simulink library "INT_ECBtn_DD"  (R2016b)
settings: Solver=VariableStepAuto  StartTime=0.0  StopTime=10.0  RelTol=1e-3
settings Model: Creator=xinchangran  LastModifiedBy=xinchangran

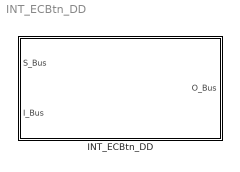
== system INT_ECBtn_DD ==
  INT_ECBtn_DD : Subsystem

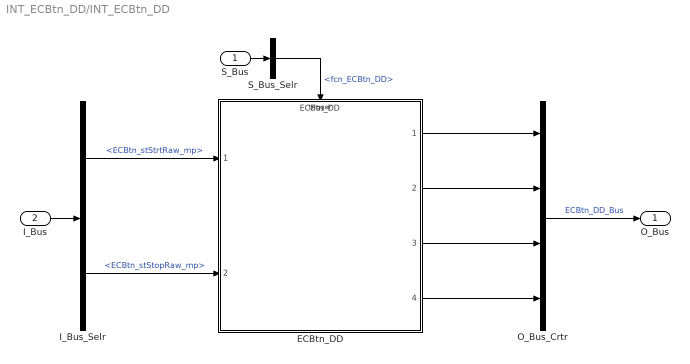
== system INT_ECBtn_DD/INT_ECBtn_DD ==
  S_Bus : Inport
  I_Bus : Inport  Port=2
  ECBtn_DD : ModelReference  ModelNameDialog=ECBtn_DD  SimulationMode=Normal  ModelReferenceVersion=1.75  TriggerPortName=function  TriggerPortTriggerType=function-call  TriggerPortStatesWhenEnabling=held
  I_Bus_Selr : BusSelector  OutputSignals=ECBtn_stStrtRaw_mp,ECBtn_stStopRaw_mp
  O_Bus_Crtr : BusCreator  Inputs=4
  S_Bus_Selr : BusSelector  OutputSignals=fcn_ECBtn_DD
  O_Bus : Outport
  wires:
  S_Bus_Selr/1 -> ECBtn_DD/Trigger  "<fcn_ECBtn_DD>"
  S_Bus/1 -> S_Bus_Selr/1
  I_Bus/1 -> I_Bus_Selr/1
  I_Bus_Selr/1 -> ECBtn_DD/1  "<ECBtn_stStrtRaw_mp>"
  I_Bus_Selr/2 -> ECBtn_DD/2  "<ECBtn_stStopRaw_mp>"
  O_Bus_Crtr/1 -> O_Bus/1  "ECBtn_DD_Bus"
  ECBtn_DD/1 -> O_Bus_Crtr/1
  ECBtn_DD/2 -> O_Bus_Crtr/2
  ECBtn_DD/3 -> O_Bus_Crtr/3
  ECBtn_DD/4 -> O_Bus_Crtr/4
